simulink model "sim_quadrotor"  (R2015a)
settings: Solver=ode3  StartTime=0  StopTime=inf  FixedStep=sampleTime_qcsim  MaxStep=0.1  RelTol=1e-3
InitFcn:
  | % load parameters of the default quadrotor
  | disp('Quadrotor parameters loaded by InitFcn')
  | paramsFilters %load mdl_quadcopter as well!
  | 
  | % change to Simulation folder if in data folder
  | cd([matlabpath '/Simulation']);
undefined symbols (not defined in the file or in its folder): altEstim, controlParams, Discrete, ofhandle, quad, quadEDT, sampleTime_qcsim, Time, vishandle
libraries: simulink x26, ctrlSharedLib x3, commnoisgen2 x1
(part 2 of 2)

== matlab function sim_quadrotor/Drone_Sensorsystem/IMU_Pressure/trafo_RTB2World_trans ==
  data: attitude input; vector input; y output
function y = fcn(attitude,vector)

yaw = attitude(1);
pitch = attitude(2);
roll = attitude(3);

R_RTBBody2Global =[ [ cos(pitch)*cos(yaw), cos(yaw)*sin(pitch)*sin(roll) - cos(roll)*sin(yaw), sin(roll)*sin(yaw) + cos(roll)*cos(yaw)*sin(pitch)];
[ cos(pitch)*sin(yaw), cos(roll)*cos(yaw) + sin(pitch)*sin(roll)*sin(yaw), cos(roll)*sin(pitch)*sin(yaw) - cos(yaw)*sin(roll)];
[         -sin(pitch),                               cos(pitch)*sin(roll),                               cos(pitch)*cos(roll)]];

% Rw_Global2RTBBody  = [0        sin(roll)          cos(roll);             %inverted Wronskian
%           0        cos(roll)*cos(pitch) -sin(roll)*cos(pitch);
%           cos(pitch) sin(roll)*sin(pitch) cos(roll)*sin(pitch)] / cos(pitch);
      
      
      
 y = R_RTBBody2Global*vector;      
      
%y = -([cos(pi/4) sin(pi/4); -sin(pi/4) cos(pi/4)]*u);

== matlab function sim_quadrotor/Drone_Sensorsystem/IMU_Pressure/trafo_World2RTB_trans1 ==
  data: attitude input; vector input; y output
function y = fcn(attitude,vector)

yaw = attitude(1);
pitch = attitude(2);
roll = attitude(3);

R_Global2RTBBody = [[                                cos(pitch)*cos(yaw),                                cos(pitch)*sin(yaw),          -sin(pitch)];
                    [ cos(yaw)*sin(pitch)*sin(roll) - cos(roll)*sin(yaw), cos(roll)*cos(yaw) + sin(pitch)*sin(roll)*sin(yaw), cos(pitch)*sin(roll)];
                    [ sin(roll)*sin(yaw) + cos(roll)*cos(yaw)*sin(pitch), cos(roll)*sin(pitch)*sin(yaw) - cos(yaw)*sin(roll), cos(pitch)*cos(roll)]];


% Rw_Global2RTBBody  = [0        sin(roll)          cos(roll);             %inverted Wronskian
%           0        cos(roll)*cos(pitch) -sin(roll)*cos(pitch);
%           cos(pitch) sin(roll)*sin(pitch) cos(roll)*sin(pitch)] / cos(pitch);
      
      
      
 y = R_Global2RTBBody*vector;      
      
%y = -([cos(pi/4) sin(pi/4); -sin(pi/4) cos(pi/4)]*u);

== matlab function sim_quadrotor/Drone_Sensorsystem/IMU_Pressure/trafo_RTB2RSSensors_rot1 ==
  data: u input; y output
function y = fcn(u)
%inverse yaw-rotation
y = [cos(pi/4)  sin(pi/4); -sin(pi/4) cos(pi/4)]*u;

== matlab function sim_quadrotor/DroneRS_Compensator/Estimator/EstimatorXYPosition/EstimatorVelocity/AccelerationWorld/World2Body ==
  data: attitude input; vector input; y output
function y = fcn(attitude,vector)

yaw = attitude(1);
pitch = attitude(2);
roll = attitude(3);

% rotz(yaw)*roty(pitch)*rotx(roll)
%     R_RTBBodytoGlobal = [cos(pitch)*cos(yaw) sin(roll)*sin(pitch)*cos(yaw)-cos(roll)*sin(yaw) cos(roll)*sin(pitch)*cos(yaw)+sin(roll)*sin(yaw);   %BBF > Inertial rotation matrix
%          cos(pitch)*sin(yaw) sin(roll)*sin(pitch)*sin(yaw)+cos(roll)*cos(yaw) cos(roll)*sin(pitch)*sin(yaw)-sin(roll)*cos(yaw);
%          -sin(pitch)         sin(roll)*cos(pitch)                            cos(roll)*cos(pitch)];
    

R_Global2RTBBody = [[                                cos(pitch)*cos(yaw),                                cos(pitch)*sin(yaw),          -sin(pitch)];
                    [ cos(yaw)*sin(pitch)*sin(roll) - cos(roll)*sin(yaw), cos(roll)*cos(yaw) + sin(pitch)*sin(roll)*sin(yaw), cos(pitch)*sin(roll)];
                    [ sin(roll)*sin(yaw) + cos(roll)*cos(yaw)*sin(pitch), cos(roll)*sin(pitch)*sin(yaw) - cos(yaw)*sin(roll), cos(pitch)*cos(roll)]];

% Rw_Global2RTBBody  = [0        sin(roll)          cos(roll);             %inverted Wronskian
%           0        cos(roll)*cos(pitch) -sin(roll)*cos(pitch);
%           cos(pitch) sin(roll)*sin(pitch) cos(roll)*sin(pitch)] / cos(pitch);
      
      
      
 y = R_Global2RTBBody*vector;      
      
%y = -([cos(pi/4) sin(pi/4); -sin(pi/4) cos(pi/4)]*u);

== matlab function sim_quadrotor/DroneRS_Compensator/Estimator/EstimatorXYPosition/EstimatorXYPosition/RStoWorld ==
  data: attitude input; vector input; vel_world output
function vel_world = fcn(attitude,vector)
yaw = attitude(1);
pitch = attitude(2);
roll = attitude(3);








R_RTBBodytoGlobal = [cos(pitch)*cos(yaw) sin(roll)*sin(pitch)*cos(yaw)-cos(roll)*sin(yaw) cos(roll)*sin(pitch)*cos(yaw)+sin(roll)*sin(yaw);   %BBF > Inertial rotation matrix
  cos(pitch)*sin(yaw) sin(roll)*sin(pitch)*sin(yaw)+cos(roll)*cos(yaw) cos(roll)*sin(pitch)*sin(yaw)-sin(roll)*cos(yaw);
  -sin(pitch)         sin(roll)*cos(pitch)                            cos(roll)*cos(pitch)];

vel_world = R_RTBBodytoGlobal*vector;

== matlab function sim_quadrotor/DroneRS_Compensator/Estimator/EstimatorAltitude/RStoWorldinacc ==
  data: attitude input; vector input; acc_world output
function acc_world = fcn(attitude,vector)
yaw = attitude(1);
pitch = attitude(2);
roll = attitude(3);








R_RTBBodytoGlobal = [cos(pitch)*cos(yaw) sin(roll)*sin(pitch)*cos(yaw)-cos(roll)*sin(yaw) cos(roll)*sin(pitch)*cos(yaw)+sin(roll)*sin(yaw);   %BBF > Inertial rotation matrix
  cos(pitch)*sin(yaw) sin(roll)*sin(pitch)*sin(yaw)+cos(roll)*cos(yaw) cos(roll)*sin(pitch)*sin(yaw)-sin(roll)*cos(yaw);
  -sin(pitch)         sin(roll)*cos(pitch)                            cos(roll)*cos(pitch)];

acc_world = R_RTBBodytoGlobal*vector;

== matlab function sim_quadrotor/DroneRS_Compensator/Estimator/EstimatorAltitude/WorldToRSinacc ==
  data: attitude input; vector input; acc_RS output
function acc_RS = fcn(attitude,vector)
yaw = attitude(1);
pitch = attitude(2);
roll = attitude(3);


R_Global2RTBBody = [[                                cos(pitch)*cos(yaw),                                cos(pitch)*sin(yaw),          -sin(pitch)];
                    [ cos(yaw)*sin(pitch)*sin(roll) - cos(roll)*sin(yaw), cos(roll)*cos(yaw) + sin(pitch)*sin(roll)*sin(yaw), cos(pitch)*sin(roll)];
                    [ sin(roll)*sin(yaw) + cos(roll)*cos(yaw)*sin(pitch), cos(roll)*sin(pitch)*sin(yaw) - cos(yaw)*sin(roll), cos(pitch)*cos(roll)]];

acc_RS = R_Global2RTBBody*vector;

== matlab function sim_quadrotor/DroneRS_Compensator/Estimator/EstimatorAttitude ==
  data: sensorIMU_datin input; yawVIS_datin input; validVIS_flagin input; gvecInit_datin input; att_estimout output; dt input; datt_estimout output; w_euler output
function [att_estimout,datt_estimout,w_euler] = fcn(sensorIMU_datin,yawVIS_datin,validVIS_flagin, gvecInit_datin,dt)
persistent yaw_cur pitch_cur roll_cur

p = sensorIMU_datin(4);
q = sensorIMU_datin(5);
r = sensorIMU_datin(6);

g = norm(gvecInit_datin,2);

if isempty(yaw_cur)
   yaw_cur = 0;
end
if isempty(pitch_cur)
   pitch_cur = 0;
end
if isempty(roll_cur)
   roll_cur = 0;
end


accvsGyro     = 0.001;
[yaw,pitch,roll,w_euler,forceMagnitudeApprox]= complimentaryfilter(yaw_cur, pitch_cur, roll_cur, g,dt,sensorIMU_datin, yawVIS_datin,validVIS_flagin,accvsGyro);
yaw_cur = yaw;
pitch_cur = pitch;
roll_cur = roll;

att_estimout = [yaw,pitch,roll]';
datt_estimout = [p,q,r]';

== matlab function sim_quadrotor/DroneRS_Compensator/Estimator/EstimatorXYPosition/EstimatorXYPosition/OutlierHandling/abs ==
  data: vec input; y output
function y = fcn(vec)
y = norm(vec,2);
